simulink library "bcm"  (R2021b)
settings: Solver=VariableStepAuto  StartTime=0.0  StopTime=10.0  RelTol=1e-3
undefined symbols (not defined in the file or in its folder): ENUM_ANTITHEFT_ALARM, ENUM_ANTITHEFT_ARM, ENUM_ANTITHEFT_DISARM, ENUM_ANTITHEFT_WAIT, ENUM_GEARPOSNTOCAN_P, ENUM_PDKEYRAWLULOCK_INUNLOCK, ENUM_PDKEYRAWPS_INPS, ENUM_POWERSTA_READY, ENUM_POWERSTA_STANDBY, FALSE, KBCM_ALMBrightnessDark_enum, KBCM_AmbBlue_enum, KBCM_AmbBreathT_K, KBCM_AmbBreathTOut_K, KBCM_AmbGreen_enum, KBCM_AmbLightUser_enum, KBCM_AmbPreset_enum, KBCM_AmbRed_enum, KBCM_Antitheft_enum_ovrdflg, KBCM_Antitheft_enum_ovrdval, KBCM_APMDoorCtrlSta_flg_ovrdflg, KBCM_APMDoorCtrlSta_flg_ovrdval, KBCM_DelayTSW_flg, KBCM_DiagFLTC_mA, KBCM_DiagFMHT_s, KBCM_DiagFRTC_mA, KBCM_DiagRLTC_mA, KBCM_DiagRRTC_mA, KBCM_DrAPMRetryTimes_cnt, KBCM_DrOpenWdwOT_s, KBCM_DrOpenWdwReady_s, KBCM_ESSOffT_ms, KBCM_ESSOnT_ms, KBCM_IVIRstHoldT_ms, KBCM_IVIRstTriggerT_ms, KBCM_ONDelayT_ms, KBCM_ReDetectT_K, KBCM_RmLampKeep_min, KBCM_RmLpKeyInT_s, KBCM_RmLpKeyMissT_s, KBCM_SlpDebounceTime_s, KBCM_SPTGDetectT_sec, KBCM_SPTGLeave_flg, KBCM_SPTGLeftBound_cm, KBCM_SPTGLeftBoundOut_cm, KBCM_SPTGLowerBound_cm, KBCM_SPTGLowerBoundOut_cm, KBCM_SPTGRightBound_cm, KBCM_SPTGRightBoundOut_cm, KBCM_SPTGTOut_K, KBCM_SPTGUpperBound_cm, KBCM_SPTGUpperBoundOut_cm, KBCM_SPTGWaitDKC_sec, KBCM_USSDis_cm, KBCM_USSFilterT_K, KBCM_WaitAPMPwr_K, KBCM_WdwManualDetT_s, MIN2SEC, TRUE, XX2KXX
libraries: simulink x41, $bdroot x3, hcu_lib x2
(part 1 of 6)
settings Model: Creator=user  LastModifiedBy=FVT22063
settings SolverCC: AlgebraicLoopSolver=TrustRegion
settings DebuggingCC: SFMachineParentedDataDiag=warning

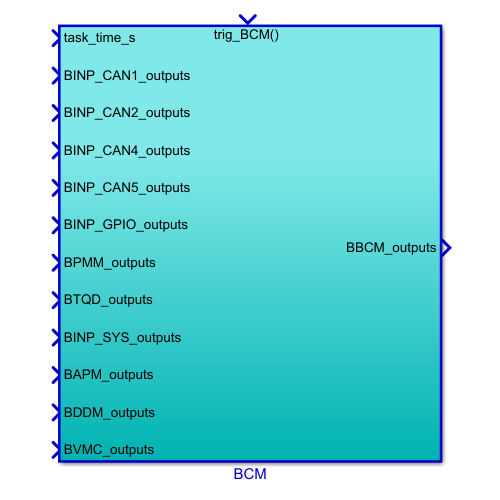
[thumbnail: Simulink's stored preview of the top-level diagram]
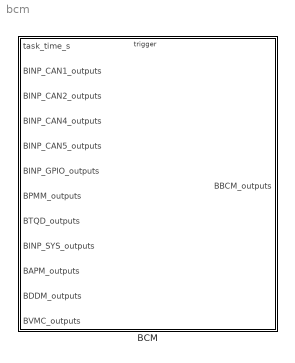
== system bcm ==
  BCM : Subsystem  TreatAsAtomicUnit=on
      settings: RTWSystemCode=Nonreusable function  RTWFcnNameOpts=Use subsystem name  RTWFileNameOpts=Use subsystem name

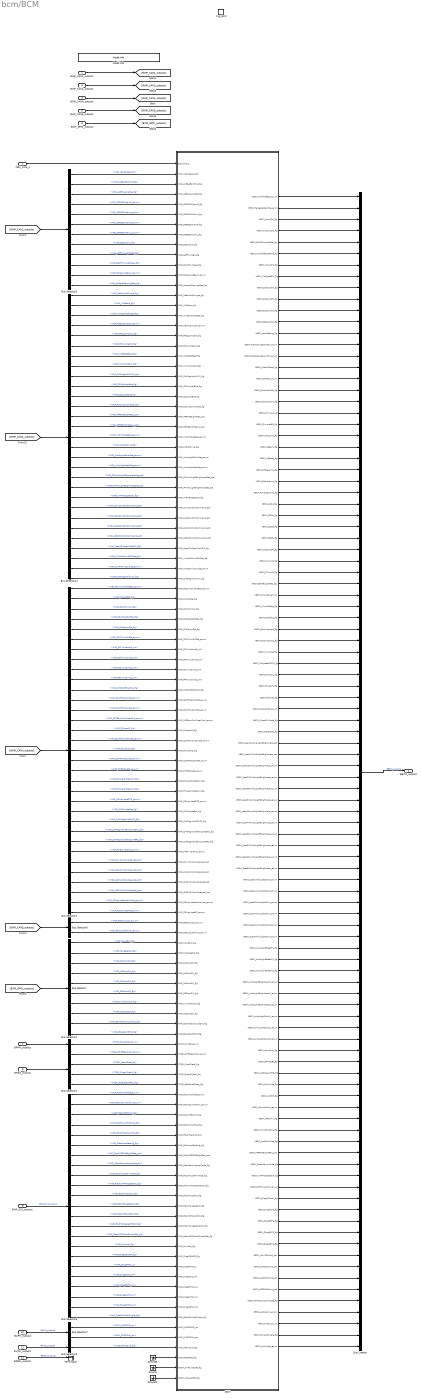
== system bcm/BCM ==
  task_time_s : Inport
  BINP_CAN1_outputs : Inport  Port=2  OutDataTypeStr=Bus: BINP_CAN1_outputs
  BINP_CAN2_outputs : Inport  Port=3  OutDataTypeStr=Bus: BINP_CAN2_outputs
  BINP_CAN4_outputs : Inport  Port=4  OutDataTypeStr=Bus: BINP_CAN4_outputs
  BINP_CAN5_outputs : Inport  Port=5  OutDataTypeStr=Bus: BINP_CAN5_outputs
  BINP_GPIO_outputs : Inport  Port=6  OutDataTypeStr=Bus: BINP_GPIO_outputs
  BPMM_outputs : Inport  Port=7  OutDataTypeStr=Bus: BPMM_outputs
  BTQD_outputs : Inport  Port=8  OutDataTypeStr=Bus: BTQD_outputs
  BINP_SYS_outputs : Inport  Port=9  OutDataTypeStr=Bus: BINP_SYS_outputs
  BAPM_outputs : Inport  Port=10  OutDataTypeStr=Bus: BAPM_outputs
  BDDM_outputs : Inport  Port=11  OutDataTypeStr=Bus: BDDM_outputs
  BVMC_outputs : Inport  Port=12  OutDataTypeStr=Bus: BVMC_outputs
  trig_BCM : TriggerPort  TriggerType=function-call  VariantControl=(inherit)
  BCM : Subsystem
  Bus Creator : BusCreator  Inputs=102  OutDataTypeStr=Bus: BBCM_outputs  NonVirtualBus=on
  Bus Selector : BusSelector  OutputSignals=VINP_HoodSW_flg,VINP_TailgateSW_flg,VINP_DrDoorSW_flg,VINP_PsDoorSW_flg,VINP_RLDoorSW_flg,VINP_RRDoorSW_flg,VINP_TrunkHanSW_flg,VINP_HazardSW_flg,VINP_CentralDoorLockSW_flg,VINP_BrakeSWGPIO_flg
  Bus Selector1 : BusSelector  OutputSignals=VPMM_PowerSta_enum
  Bus Selector14 : BusSelector  OutputSignals=VINP_SetUnlockSingle_flg,VINP_IVIStatus_flg,VINP_IVINightModeSta_flg,VINP_HeadLampSW_enum,VINP_RFogLampSW_flg,VINP_FollowMeSW_flg,VINP_IVIRRDefReq_flg,VINP_IVIWIMAINSW_flg,VINP_CANMsgValidIVI2_flg,VINP_CDLUnlockButt_flg,VINP_CDLLockButt_flg,VINP_RoomLampMode_flg,VINP_MFRDNBrightReq_pct,VINP_METERKPHCalcu_kph,VINP_IVIPWModeReq_enum,VINP_LINKtoDrive_flg,VINP_AmbLightColorSet_enum,VINP_AmbLightUserSet_enum,VINP_DRAmbLightBrightnessSet_pct,VINP_IPAmbLightBrightnessSet_pct,VINP_IVIPTGUSStaSW_flg,VINP_LDrvControlCommand_pct,VINP_LPasControlCommand_pct,VINP_LRLDControlCommand_pct,VINP_LRRDControlCommand_pct,VINP_OpenDrOpenWdoSW_flg,VINP_IVILockSoundSWSta_flg,VINP_AVMParkingmode_enum,VINP_CANMsgValidIVI1_flg
  Bus Selector2 : BusSelector  OutputSignals=VINP_PCommandToBCM_enum,VINP_DrLockSta_flg,VINP_CSWDimSw_flg,VINP_CSWPassSWSta_flg,VINP_RLSLampSta_flg,VINP_CSWTurnSwSta_enum,VINP_RLTurnLampC_mA,VINP_RRTurnLampC_mA,VINP_FLTurnLampC_mA,VINP_FRTurnLampC_mA,VINP_MIRRORFOLDSW_flg,VINP_CSWFWasSwSta_enum,VINP_CSWFWipSwSta_enum,VINP_RLSRainSnrWiperCmd_enum,VINP_FWiperAS_flg,VINP_CSWRWipIntSwSta_enum,VINP_RWiperAS_flg,VINP_CSWRWasSWSta_enum,VINP_PTGRDILSta_enum,VINP_RWiperProtection_flg,VINP_FWiperProtection_flg,VINP_PDKeyAreaPTG_enum,VINP_SWCmodeSta_flg,VINP_CANMsgValidDKC1_flg,VINP_CANMsgValidGWZoneDR1_flg,VINP_CANMsgValidGWZoneFR1_flg,VINP_PTGInnerSW2_enum,VINP_LDrvValWdwOpened_pct,VINP_LPasValWdwOpened_pct,VINP_LRLDValWdwOpened_pct,VINP_LRRDValWdwOpened_pct,VINP_PDKeyAreaLockUnlock_enum,VINP_PDKeyAreaPS_enum
  Bus Selector3 : BusSelector  OutputSignals=VINP_VehSpeed_kph,VINP_AirBagFailCmd_flg,VINP_ActBrkLampSta_flg,VINP_SRRODAWarnR_enum,VINP_SRRODAWarnL_enum,VINP_SRRBSDWarnR_enum,VINP_SRRBSDWarnL_enum,VINP_ESSActive_flg,VINP_LeftTurnLightReq_flg,VINP_RightTurnLightReq_flg,VINP_ForceLowBeam_enum,VINP_HazardWarningReq_flg
  Bus Selector4 : BusSelector  OutputSignals=VTQD_ShiftGearPosn_enum,VTQD_CrashDetd_flg,VTQD_DiagHCrash_flg,VTQD_ReBrakeLPReq_flg
  Bus Selector5 : BusSelector  OutputSignals=VINP_ReDoorLock_enum,VINP_ReOutsideMirror_enum
  Bus Selector6 : BusSelector  OutputSignals=VINP_FlashAntitheft_enum,VINP_FlashCountAlarm_enum,VINP_FlashMFSWTri_flg,VINP_FlashMirrorFlodPos_flg,VINP_FlashFuelDoorPos_flg,VINP_FlashLockSetting_flg,VINP_FlashMFRDNBrightReq_pct,VINP_FlashRoomLampMode_flg,VINP_FlashWiperFixMode_flg,VINP_FlashIVIPTGUSStaSW_flg,VINP_FlashHoodSW_flg,VINP_FlashTailgateSW_flg,VINP_FlashCTDLockSW_flg,VINP_FlashTailgateHDSW_flg,VINP_FlashAPMDoorControlSta_flg,VINP_funAuto_flg,VINP_DiagDRLOFF_flg,VINP_DiagFMHT_s,VINP_DiagFLTC_mA,VINP_DiagFRTC_mA,VINP_DiagRLTC_mA,VINP_DiagRRTC_mA,VINP_FlashfUnlockSingle_flg
  Bus Selector7 : BusSelector  OutputSignals=VAPM_PASDRMR_cm,VAPM_PASDRML_cm
  Bus Selector8 : BusSelector  OutputSignals=VVMC_APSActive_flg
  Ground : Ground
  Ground1 : Ground
  Ground6 : Ground
  Model Info : simulink/Model-Wide Utilities/Model Info  Frame=on  DisplayStringWithTags=$Id: pmm.mdl 130 2021-02-08 12:40:01Z Shawn $  HorizontalTextAlignment=Center  LeftAlignmentValue=0.5
  Terminator : Terminator
  BBCM_outputs : Outport  OutDataTypeStr=Bus: BBCM_outputs  VectorParamsAs1DForOutWhenUnconnected=off
  wires:
  Bus Creator/1 -> BBCM_outputs/1  "BBCM_outputs"
  BPMM_outputs/1 -> Bus Selector1/1
  BINP_CAN4_outputs/1 -> [BINP_CAN4_outputs]
  BINP_CAN1_outputs/1 -> [BINP_CAN1_outputs]
  [BINP_CAN1_outputs] -> Bus Selector3/1
  BINP_GPIO_outputs/1 -> [BINP_GPIO_outputs]
  [BINP_GPIO_outputs] -> Bus Selector/1
  BINP_CAN2_outputs/1 -> [BINP_CAN2_outputs]
  BINP_CAN5_outputs/1 -> [BINP_CAN5_outputs]
  [BINP_CAN2_outputs] -> Bus Selector14/1
  Bus Selector/1 -> BCM/78(VINP_HoodSW_flg)  "<VINP_HoodSW_flg>"
  Bus Selector/2 -> BCM/79(VINP_TailgateSW_flg)  "<VINP_TailgateSW_flg>"
  Bus Selector/3 -> BCM/80(VINP_DrDoorSW_flg)  "<VINP_DrDoorSW_flg>"
  Bus Selector/4 -> BCM/81(VINP_PsDoorSW_flg)  "<VINP_PsDoorSW_flg>"
  Bus Selector/5 -> BCM/82(VINP_RLDoorSW_flg)  "<VINP_RLDoorSW_flg>"
  Bus Selector/6 -> BCM/83(VINP_RRDoorSW_flg)  "<VINP_RRDoorSW_flg>"
  Bus Selector/7 -> BCM/84(VINP_TrunkHanSW_flg)  "<VINP_TrunkHanSW_flg>"
  Bus Selector/8 -> BCM/85(VINP_HazardSW_flg)  "<VINP_HazardSW_flg>"
  Bus Selector1/1 -> BCM/88(VPMM_PwrSta_enum)  "<VPMM_PowerSta_enum>"
  Bus Selector/9 -> BCM/86(VINP_CentralDoorLockSW_flg)  "<VINP_CentralDoorLockSW_flg>"
  Bus Selector4/1 -> BCM/89(VTQD_ShiftGearPosn_enum)  "<VTQD_ShiftGearPosn_enum>"
  BTQD_outputs/1 -> Bus Selector4/1
  Bus Selector3/2 -> BCM/3(VINP_AirBagFailCmd_flg)  "<VINP_AirBagFailCmd_flg>"
  Bus Selector3/3 -> BCM/4(VINP_ActBrkLampSta_flg)  "<VINP_ActBrkLampSta_flg>"
  Bus Selector3/1 -> BCM/2(VINP_VehSpeed_kph)  "<VINP_VehSpeed_kph>"
  Bus Selector3/4 -> BCM/5(VINP_SRRODAWarnR_flg)  "<VINP_SRRODAWarnR_enum>"
  Bus Selector3/5 -> BCM/6(VINP_SRRODAWarnL_flg)  "<VINP_SRRODAWarnL_enum>"
  Bus Selector3/6 -> BCM/7(VINP_SRRBSDWarnR_flg)  "<VINP_SRRBSDWarnR_enum>"
  Bus Selector3/7 -> BCM/8(VINP_SRRBSDWarnL_flg)  "<VINP_SRRBSDWarnL_enum>"
  Bus Selector3/8 -> BCM/9(VINP_ESSActive_flg)  "<VINP_ESSActive_flg>"
  Bus Selector3/9 -> BCM/10(VINP_LeftTurnReq_flg)  "<VINP_LeftTurnLightReq_flg>"
  Bus Selector3/10 -> BCM/11(VINP_RightTurnReq_flg)  "<VINP_RightTurnLightReq_flg>"
  Bus Selector3/11 -> BCM/12(VINP_ForceLowBeam_enum)  "<VINP_ForceLowBeam_enum>"
  [BINP_CAN4_outputs] -> Bus Selector2/1
  Bus Selector2/1 -> BCM/43(VINP_PCommandToBCM_enum)  "<VINP_PCommandToBCM_enum>"
  Bus Selector2/2 -> BCM/44(VINP_DrLockSta_flg)  "<VINP_DrLockSta_flg>"
  Bus Selector2/3 -> BCM/45(VINP_CSWDimSw_flg)  "<VINP_CSWDimSw_flg>"
  Bus Selector2/4 -> BCM/46(VINP_CSWPassSWSta_flg)  "<VINP_CSWPassSWSta_flg>"
  Bus Selector2/5 -> BCM/47(VINP_RLSLampSta_flg)  "<VINP_RLSLampSta_flg>"
  Bus Selector2/6 -> BCM/48(VINP_CSWTurnSWSta_enum)  "<VINP_CSWTurnSwSta_enum>"
  Bus Selector2/7 -> BCM/49(VINP_RLTurnLampC_mA)  "<VINP_RLTurnLampC_mA>"
  Bus Selector2/8 -> BCM/50(VINP_RRTurnLampC_mA)  "<VINP_RRTurnLampC_mA>"
  Bus Selector2/9 -> BCM/51(VINP_FLTurnLampC_mA)  "<VINP_FLTurnLampC_mA>"
  Bus Selector2/10 -> BCM/52(VINP_FRTurnLampC_mA)  "<VINP_FRTurnLampC_mA>"
  Bus Selector2/11 -> BCM/53(VINP_MIRRORFOLDSW_flg)  "<VINP_MIRRORFOLDSW_flg>"
  Bus Selector2/12 -> BCM/54(VINP_CSWFWasSWSta_enum)  "<VINP_CSWFWasSwSta_enum>"
  Bus Selector2/13 -> BCM/55(VINP_CSWFWipSWSta_enum)  "<VINP_CSWFWipSwSta_enum>"
  Bus Selector2/14 -> BCM/56(VINP_RLSRainSnrWiperCmd_enum)  "<VINP_RLSRainSnrWiperCmd_enum>"
  Bus Selector2/15 -> BCM/57(VINP_FWiperAS_flg)  "<VINP_FWiperAS_flg>"
  Bus Selector2/16 -> BCM/58(VINP_CSWRWipIntSwSta_enum)  "<VINP_CSWRWipIntSwSta_enum>"
  Bus Selector2/17 -> BCM/59(VINP_RWiperAS_flg)  "<VINP_RWiperAS_flg>"
  Bus Selector2/18 -> BCM/60(VINP_CSWRWasSWSta_enum)  "<VINP_CSWRWasSWSta_enum>"
  [BINP_CAN5_outputs] -> Bus Selector5/1
  Bus Selector5/1 -> BCM/76(VINP_ReDoorLock_enum)  "<VINP_ReDoorLock_enum>"
  Bus Selector14/9 -> BCM/22(VINP_CANMsgValidIVI2_flg)  "<VINP_CANMsgValidIVI2_flg>"
  Ground6/1 -> BCM/119(VINP_RRDefSta_flg)
  Bus Selector14/2 -> BCM/15(VINP_IVIStatus_flg)  "<VINP_IVIStatus_flg>"
  Bus Selector14/3 -> BCM/16(VINP_IVINightModeSta_flg)  "<VINP_IVINightModeSta_flg>"
  Bus Selector14/4 -> BCM/17(VINP_HeadLampSW_enum)  "<VINP_HeadLampSW_enum>"
  Bus Selector14/5 -> BCM/18(VINP_RFogLampSW_flg)  "<VINP_RFogLampSW_flg>"
  Bus Selector14/6 -> BCM/19(VINP_FollowMeSW_flg)  "<VINP_FollowMeSW_flg>"
  Bus Selector14/1 -> BCM/14(VINP_SetUnlockSingle_flg)  "<VINP_SetUnlockSingle_flg>"
  Bus Selector14/7 -> BCM/20(VINP_IVIRRDefReq_flg)  "<VINP_IVIRRDefReq_flg>"
  Bus Selector14/8 -> BCM/21(VINP_IVIWIMAINSW_flg)  "<VINP_IVIWIMAINSW_flg>"
  Bus Selector14/10 -> BCM/23(VINP_CDLUnlockButt_flg)  "<VINP_CDLUnlockButt_flg>"
  Bus Selector14/11 -> BCM/24(VINP_CDLLockButt_flg)  "<VINP_CDLLockButt_flg>"
  Bus Selector14/12 -> BCM/25(VINP_RoomLampMode_flg)  "<VINP_RoomLampMode_flg>"
  Bus Selector2/19 -> BCM/61(VINP_PTGRDILsta_enum)  "<VINP_PTGRDILSta_enum>"
  Bus Selector3/12 -> BCM/13(VINP_HazardWarningReq_flg)  "<VINP_HazardWarningReq_flg>"
  Bus Selector/10 -> BCM/87(VINP_BrakeSWGPIO_flg)  "<VINP_BrakeSWGPIO_flg>"
  Bus Selector14/13 -> BCM/26(VINP_MFRDNBrightReq_pct)  "<VINP_MFRDNBrightReq_pct>"
  Bus Selector4/2 -> BCM/90(VTQD_CrashDetd_flg)  "<VTQD_CrashDetd_flg>"
  Bus Selector4/3 -> BCM/91(VTQD_DiagHCrash_flg)  "<VTQD_DiagHCrash_flg>"
  Bus Selector4/4 -> BCM/92(VTQD_ReBrakeLPReq_flg)  "<VTQD_ReBrakeLPReq_flg>"
  Bus Selector14/14 -> BCM/27(VINP_METERKPHCalcu_kph)  "<VINP_METERKPHCalcu_kph>"
  Bus Selector14/15 -> BCM/28(VINP_IVIPWModeReq_enum)  "<VINP_IVIPWModeReq_enum>"
  task_time_s/1 -> BCM/1(task_time_s)
  Bus Selector14/16 -> BCM/29(VINP_LINKtoDrive_flg)  "<VINP_LINKtoDrive_flg>"
  Bus Selector5/2 -> BCM/77(VINP_ReOutsideMirror_enum)  "<VINP_ReOutsideMirror_enum>"
  Bus Selector14/17 -> BCM/30(VINP_AmbLightColorSet_enum)  "<VINP_AmbLightColorSet_enum>"
  Bus Selector14/18 -> BCM/31(VINP_AmbLightUserSet_enum)  "<VINP_AmbLightUserSet_enum>"
  Bus Selector14/19 -> BCM/32(VINP_DRAmbLightBrightnessSet_pct)  "<VINP_DRAmbLightBrightnessSet_pct>"
  Bus Selector14/20 -> BCM/33(VINP_IPAmbLightBrightnessSet_pct)  "<VINP_IPAmbLightBrightnessSet_pct>"
  BINP_SYS_outputs/1 -> Bus Selector6/1  "BINP_SYS_output"
  Bus Selector6/1 -> BCM/93(VINP_FlashAntitheft_enum)  "<VINP_FlashAntitheft_enum>"
  Bus Selector2/21 -> BCM/63(VINP_FWiperProtection_flg)  "<VINP_FWiperProtection_flg>"
  Bus Selector2/20 -> BCM/62(VINP_RWiperProtection_flg)  "<VINP_RWiperProtection_flg>"
  Bus Selector2/22 -> BCM/64(VINP_PDKeyAreaPTG_enum)  "<VINP_PDKeyAreaPTG_enum>"
  Bus Selector14/21 -> BCM/34(VINP_IVIPTGUSStaSW_flg)  "<VINP_IVIPTGUSStaSW_flg>"
  BAPM_outputs/1 -> Bus Selector7/1  "BAPM_outputs"
  Bus Selector7/1 -> BCM/116(VAPM_PASDRMR_cm)  "<VAPM_PASDRMR_cm>"
  Bus Selector7/2 -> BCM/117(VAPM_PASDRML_cm)  "<VAPM_PASDRML_cm>"
  Bus Selector2/24 -> BCM/66(VINP_CANMsgValidDKC1_flg)  "<VINP_CANMsgValidDKC1_flg>"
  Bus Selector2/23 -> BCM/65(VINP_SWCmodeSta_flg)  "<VINP_SWCmodeSta_flg>"
  Bus Selector2/25 -> BCM/67(VINP_CANMsgValidGWZoneDR1_flg)  "<VINP_CANMsgValidGWZoneDR1_flg>"
  Bus Selector2/26 -> BCM/68(VINP_CANMsgValidGWZoneFR1_flg)  "<VINP_CANMsgValidGWZoneFR1_flg>"
  Bus Selector6/2 -> BCM/94(VINP_FlashCountAlarm_enum)  "<VINP_FlashCountAlarm_enum>"
  Bus Selector6/3 -> BCM/95(VINP_FlashMFSWTri_flg)  "<VINP_FlashMFSWTri_flg>"
  Bus Selector6/4 -> BCM/96(VINP_FlashMirrorFlodPos)  "<VINP_FlashMirrorFlodPos_flg>"
  Bus Selector6/5 -> BCM/97(VINP_FlashFuelDoorPos)  "<VINP_FlashFuelDoorPos_flg>"
  Bus Selector6/6 -> BCM/98(VINP_FlashLockSetting_flg)  "<VINP_FlashLockSetting_flg>"
  Bus Selector6/7 -> BCM/99(VINP_FlashMFRDNBrightReq_pct)  "<VINP_FlashMFRDNBrightReq_pct>"
  Bus Selector6/8 -> BCM/100(VINP_FlashRoomLampMode_flg)  "<VINP_FlashRoomLampMode_flg>"
  Bus Selector6/9 -> BCM/101(VINP_FlashWiperFixMode_flg)  "<VINP_FlashWiperFixMode_flg>"
  Bus Selector6/10 -> BCM/102(VINP_FlashIVIPTGUSStaSW_flg)  "<VINP_FlashIVIPTGUSStaSW_flg>"
  Bus Selector2/27 -> BCM/69(VINP_PTGInnerSW2_enum)  "<VINP_PTGInnerSW2_enum>"
  BCM/1(VBCM_AntitheftSta_enum) -> Bus Creator/1
  BCM/2(VBCM_TailgateRemote_enum) -> Bus Creator/2
  BCM/3(VBCM_HornCtrl_flg) -> Bus Creator/3
  BCM/4(VBCM_AllDoorSW_flg) -> Bus Creator/4
  BCM/5(VBCM_BCMDoorLockSta_flg) -> Bus Creator/5
  BCM/6(VBCM_AntitheftSeatFlod_flg) -> Bus Creator/6
  BCM/7(VBCM_HoodSW_flg) -> Bus Creator/7
  BCM/8(VBCM_TailgateSW_flg) -> Bus Creator/8
  BCM/9(VBCM_DrDoorSW_flg) -> Bus Creator/9
  BCM/10(VBCM_PsDoorSW_flg) -> Bus Creator/10
  BCM/11(VBCM_RLDoorSW_flg) -> Bus Creator/11
  BCM/12(VBCM_RRDoorSW_flg) -> Bus Creator/12
  BCM/13(VBCM_LockSetting_flg) -> Bus Creator/13
  BCM/14(VBCM_FrChargingDoorCtrl_enum) -> Bus Creator/14
  BCM/15(VBCM_RrChargingDoorCtrl_enum) -> Bus Creator/15
  BCM/16(VBCM_CrashSDetd_flg) -> Bus Creator/16
  BCM/17(VBCM_CTDCtrl_enum) -> Bus Creator/17
  BCM/18(VBCM_DoorLockIND_flg) -> Bus Creator/18
  BCM/19(VBCM_CTDLockSW_flg) -> Bus Creator/19
  BCM/20(VBCM_Dimmer_pct) -> Bus Creator/20
  BCM/21(VBCM_DimmerEN_flg) -> Bus Creator/21
  BCM/22(VBCM_PosLamp_flg) -> Bus Creator/22
  BCM/23(VBCM_LBeam_flg) -> Bus Creator/23
  BCM/24(VBCM_HBeam_flg) -> Bus Creator/24
  BCM/25(VBCM_RrFogLamp_flg) -> Bus Creator/25
  BCM/26(VBCM_BrakeLamp_flg) -> Bus Creator/26
  BCM/27(VBCM_ReverseLamp_flg) -> Bus Creator/27
  BCM/28(VBCM_LDRL_flg) -> Bus Creator/28
  BCM/29(VBCM_RDRL_flg) -> Bus Creator/29
  BCM/30(VBCM_LBSD_flg) -> Bus Creator/30
  BCM/31(VBCM_RBSD_flg) -> Bus Creator/31
  BCM/32(VBCM_HazardSW_flg) -> Bus Creator/32
  BCM/33(VBCM_LTurnLP_flg) -> Bus Creator/33
  BCM/34(VBCM_RTurnLP_flg) -> Bus Creator/34
  BCM/35(VBCM_BCMBuzzerReq_flg) -> Bus Creator/35
  BCM/36(VBCM_MirrorCtrl_enum) -> Bus Creator/36
  BCM/37(VBCM_MirrorDefog_flg) -> Bus Creator/37
  BCM/38(VBCM_RrDefog_flg) -> Bus Creator/38
  BCM/39(VBCM_RoomLampH_flg) -> Bus Creator/39
  BCM/40(VBCM_RoomLampL_flg) -> Bus Creator/40
  BCM/41(VBCM_TrunkRel_flg) -> Bus Creator/41
  BCM/42(VBCM_TailgateHDSW_flg) -> Bus Creator/42
  BCM/43(VBCM_FWiperL_flg) -> Bus Creator/43
  BCM/44(VBCM_FWiperH_flg) -> Bus Creator/44
  BCM/45(VBCM_RWiper_flg) -> Bus Creator/45
  BCM/46(VBCM_WasherCtrl_enum) -> Bus Creator/46
  BCM/47(VBCM_WiperFixMode_flg) -> Bus Creator/47
  BCM/48(VBCM_SleepReq_flg) -> Bus Creator/48
  BCM/49(VBCM_User1DrAmbLightBrightness_pct) -> Bus Creator/49
  BCM/50(VBCM_User1IPAmbLightBrightness_pct) -> Bus Creator/50
  BCM/51(VBCM_User2DrAmbLightBrightness_enum) -> Bus Creator/51
  BCM/52(VBCM_User2IPAmbLightBrightness_enum) -> Bus Creator/52
  BCM/53(VBCM_User3DrAmbLightBrightness_enum) -> Bus Creator/53
  BCM/54(VBCM_User3IPAmbLightBrightness_enum) -> Bus Creator/54
  BCM/55(VBCM_User4DrAmbLightBrightness_enum) -> Bus Creator/55
  BCM/56(VBCM_User4IPAmbLightBrightness_enum) -> Bus Creator/56
  BCM/57(VBCM_User5DrAmbLightBrightness_enum) -> Bus Creator/57
  BCM/58(VBCM_User5IPAmbLightBrightness_enum) -> Bus Creator/58
  BCM/59(VBCM_User6DrAmbLightBrightness_enum) -> Bus Creator/59
  BCM/60(VBCM_User6IPAmbLightBrightness_enum) -> Bus Creator/60
  BCM/61(VBCM_User1AmbLightColor_enum) -> Bus Creator/61
  BCM/62(VBCM_User2AmbLightColor_enum) -> Bus Creator/62
  BCM/63(VBCM_User3AmbLightColor_enum) -> Bus Creator/63
  BCM/64(VBCM_User4AmbLightColor_enum) -> Bus Creator/64
  BCM/65(VBCM_User5AmbLightColor_enum) -> Bus Creator/65
  BCM/66(VBCM_User6AmbLightColor_enum) -> Bus Creator/66
  BCM/67(VBCM_AmbLightBreath1_flg) -> Bus Creator/67
  BCM/68(VBCM_AmbLightBreath2_flg) -> Bus Creator/68
  BCM/69(VBCM_AmbLightBreath3_flg) -> Bus Creator/69
  BCM/70(VBCM_AmbLightBrightness1_enum) -> Bus Creator/70
  BCM/71(VBCM_AmbLightBrightness2_enum) -> Bus Creator/71
  BCM/72(VBCM_AmbLightBrightness3_enum) -> Bus Creator/72
  BCM/73(VBCM_AmbLightColor1_enum) -> Bus Creator/73
  BCM/74(VBCM_AmbLightColor2_enum) -> Bus Creator/74
  BCM/75(VBCM_AmbLightColor3_enum) -> Bus Creator/75
  BCM/76(VBCM_LampPwr_flg) -> Bus Creator/76
  BCM/77(VBCM_SPTGDet_flg) -> Bus Creator/77
  BCM/78(VBCM_APSOpenPTG_flg) -> Bus Creator/78
  BCM/79(VBCM_FollowMe_flg) -> Bus Creator/79
  BCM/80(VBCM_IVIRST_flg) -> Bus Creator/80
  BCM/81(VBCM_CountAlarm_enum) -> Bus Creator/81
  BCM/82(VBCM_MFSWTri_flg) -> Bus Creator/82
  BCM/83(VBCM_MirrorFlodPos_flg) -> Bus Creator/83
  BCM/84(VBCM_FuelDoorPos_flg) -> Bus Creator/84
  BCM/85(VBCM_MFRDNBrightReq_pct) -> Bus Creator/85
  BCM/86(VBCM_RoomLampMode_flg) -> Bus Creator/86
  BCM/87(VBCM_IVIPTGUSStaSW_flg) -> Bus Creator/87
  BCM/88(VBCM_PTGInnerSW2_enum) -> Bus Creator/88
  BCM/89(VBCM_DiagHCrash_flg) -> Bus Creator/89
  BCM/90(VBCM_DiagFLTS_flg) -> Bus Creator/90
  BCM/91(VBCM_DiagFRTS_flg) -> Bus Creator/91
  BCM/92(VBCM_DiagRLTS_flg) -> Bus Creator/92
  BCM/93(VBCM_DiagRRTS_flg) -> Bus Creator/93
  Bus Selector6/11 -> BCM/103(VINP_FlashHoodSW_flg)  "<VINP_FlashHoodSW_flg>"
  Bus Selector6/12 -> BCM/104(VINP_FlashTailgateSW_flg)  "<VINP_FlashTailgateSW_flg>"
  Bus Selector6/13 -> BCM/105(VINP_FlashCTDLockSW_flg)  "<VINP_FlashCTDLockSW_flg>"
  Bus Selector6/14 -> BCM/106(VINP_FlashTailgateHDSW_flg)  "<VINP_FlashTailgateHDSW_flg>"
  BCM/94(VBCM_LDrvCtrlCmd_pct) -> Bus Creator/94
  BCM/95(VBCM_LPasCtrlCmd_pct) -> Bus Creator/95
  BCM/96(VBCM_LRLDCtrlCmd_pct) -> Bus Creator/96
  BCM/97(VBCM_LRRDCtrlCmd_pct) -> Bus Creator/97
  BCM/98(VBCM_APMDoorControlSta_flg) -> Bus Creator/98
  Bus Selector14/25 -> BCM/38(VINP_LRRDControlCommand_pct)  "<VINP_LRRDControlCommand_pct>"
  Bus Selector14/24 -> BCM/37(VINP_LRLDControlCommand_pct)  "<VINP_LRLDControlCommand_pct>"
  Bus Selector14/23 -> BCM/36(VINP_LPasControlCommand_pct)  "<VINP_LPasControlCommand_pct>"
  Bus Selector14/22 -> BCM/35(VINP_LDrvControlCommand_pct)  "<VINP_LDrvControlCommand_pct>"
  Bus Selector2/28 -> BCM/70(VINP_LDrvValWdwOpened_pct)  "<VINP_LDrvValWdwOpened_pct>"
  Bus Selector2/29 -> BCM/71(VINP_LPasValWdwOpened_pct)  "<VINP_LPasValWdwOpened_pct>"
  Bus Selector2/30 -> BCM/72(VINP_LRLDValWdwOpened_pct)  "<VINP_LRLDValWdwOpened_pct>"
  Bus Selector2/31 -> BCM/73(VINP_LRRDValWdwOpened_pct)  "<VINP_LRRDValWdwOpened_pct>"
  Bus Selector14/26 -> BCM/39(VINP_OpenDrOpenWdoSW_flg)  "<VINP_OpenDrOpenWdoSW_flg>"
  Bus Selector6/15 -> BCM/107(VINP_FlashAPMDoorControlSta_flg)  "<VINP_FlashAPMDoorControlSta_flg>"
  Ground/1 -> BCM/120(VDDM_HVRlyOpCFS_flg)
  Ground1/1 -> BCM/121(VDDM_MCUActCFS_flg)
  BDDM_outputs/1 -> Terminator/1  "BDDM_outputs"
  Bus Selector2/32 -> BCM/74(VINP_PDKeyAreaLockUnlock_enum)  "<VINP_PDKeyAreaLockUnlock_enum>"
  Bus Selector2/33 -> BCM/75(VINP_PDKeyAreaPS_enum)  "<VINP_PDKeyAreaPS_enum>"
  Bus Selector14/27 -> BCM/40(VINP_IVILockSoundSWSta_flg)  "<VINP_IVILockSoundSWSta_flg>"
  Bus Selector6/16 -> BCM/108(VINP_funAuto_flg)  "<VINP_funAuto_flg>"
  Bus Selector6/17 -> BCM/109(VINP_DiagDRLOFF_flg)  "<VINP_DiagDRLOFF_flg>"
  Bus Selector6/18 -> BCM/110(VINP_DiagFMHT_s)  "<VINP_DiagFMHT_s>"
  Bus Selector6/19 -> BCM/111(VINP_DiagFLTC_mA)  "<VINP_DiagFLTC_mA>"
  Bus Selector6/20 -> BCM/112(VINP_DiagFRTC_mA)  "<VINP_DiagFRTC_mA>"
  Bus Selector6/21 -> BCM/113(VINP_DiagRLTC_mA)  "<VINP_DiagRLTC_mA>"
  Bus Selector6/22 -> BCM/114(VINP_DiagRRTC_mA)  "<VINP_DiagRRTC_mA>"
  BVMC_outputs/1 -> Bus Selector8/1  "BVMC_outputs"
  Bus Selector8/1 -> BCM/118(VINP_APSActive_flg)  "<VVMC_APSActive_flg>"
  Bus Selector14/28 -> BCM/41(VINP_AVMparkingmode_enum)  "<VINP_AVMParkingmode_enum>"
  Bus Selector14/29 -> BCM/42(VINP_CANMsgValidIVI1_flg)  "<VINP_CANMsgValidIVI1_flg>"
  BCM/99(VBCM_LockAlarm_enum) -> Bus Creator/99
  BCM/100(VBCM_ATCtrl_enum) -> Bus Creator/100
  BCM/101(VBCM_fUnlockSingle_flg) -> Bus Creator/101
  Bus Selector6/23 -> BCM/115(VINP_FlashfUnlockSingle_flg)  "<VINP_FlashfUnlockSingle_flg>"
  BCM/102(VBCM_OutMode_enum) -> Bus Creator/102
